simulink model "problem2_4"  (R2020a)
settings: Solver=VariableStepAuto  StartTime=0.0  StopTime=10.0  RelTol=1e-3
settings Model: EnablePacing=on  PacingRate=110  Creator=dinhm  LastModifiedBy=dinhm

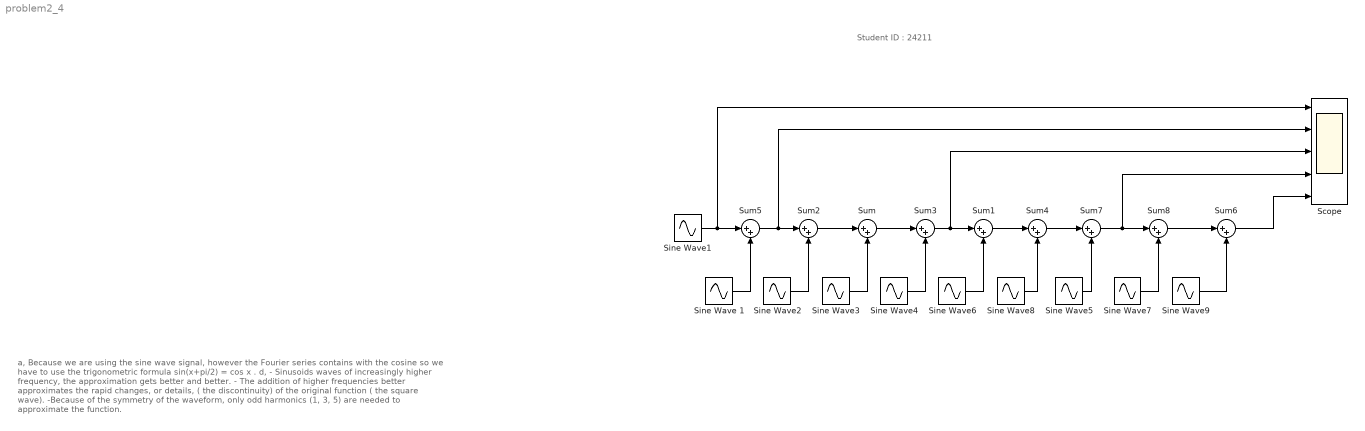
== system problem2_4 ==
  note: a, Because we are using the sine wave signal, however the Fourier series contains with the cosine so we have to use the trigonometric formula sin(x+pi/2) = cos x .
      |
      | d,
      | - Sinusoids waves of increasingly higher frequency, the approximation gets better and better.
      | - The addition of higher frequencies better approximates the rapid changes, or details, ( the discontinuity) of the original function ( the square wave).
      | -Because of the symmetry of the waveform, only odd harmonics (1, 3, 5) are needed to approximate the function.
  note: Student ID : 24211
  Scope : Scope  NumInputPorts=5
  Sine Wave 1 : Sin  Amplitude=4/pi*(-1/3)  Frequency=3*(2*pi/11)  Phase=pi/2  SampleTime=0.1
  Sine Wave1 : Sin  Amplitude=4/pi*1  Frequency=1*(2*pi/11)  Phase=pi/2  SampleTime=0.1
  Sine Wave2 : Sin  Amplitude=4/pi*(1/5)  Frequency=5*(2*pi/11)  Phase=pi/2  SampleTime=0.1
  Sine Wave3 : Sin  Amplitude=4/pi*(-1/7)  Frequency=7*(2*pi/11)  Phase=pi/2  SampleTime=0.1
  Sine Wave4 : Sin  Amplitude=4/pi*(1/9)  Frequency=9*(2*pi/11)  Phase=pi/2  SampleTime=0.1
  Sine Wave5 : Sin  Amplitude=4/pi*(-1/15)  Frequency=15*(2*pi/11)  Phase=pi/2  SampleTime=0.1
  Sine Wave6 : Sin  Amplitude=4/pi*(-1/11)  Frequency=11*(2*pi/11)  Phase=pi/2  SampleTime=0.1
  Sine Wave7 : Sin  Amplitude=4/pi*(1/17)  Frequency=17*(2*pi/11)  Phase=pi/2  SampleTime=0.1
  Sine Wave8 : Sin  Amplitude=4/pi*(1/13)  Frequency=13*(2*pi/11)  Phase=pi/2  SampleTime=0.1
  Sine Wave9 : Sin  Amplitude=4/pi*(-1/19)  Frequency=19*(2*pi/11)  Phase=pi/2  SampleTime=0.1
  Sum{,1..8} (9 alike) : Sum  Inputs=|++
  wires:
  Sine Wave9/1 -> Sum6/2
  Sine Wave7/1 -> Sum8/2
  Sine Wave5/1 -> Sum7/2
  Sine Wave8/1 -> Sum4/2
  Sine Wave6/1 -> Sum1/2
  Sine Wave4/1 -> Sum3/2
  Sine Wave3/1 -> Sum/2
  Sine Wave2/1 -> Sum2/2
  Sum2/1 -> Sum/1
  Sum/1 -> Sum3/1
  Sum1/1 -> Sum4/1
  Sum4/1 -> Sum7/1
  Sum7/1 -> Scope/4, Sum8/1
  Sum8/1 -> Sum6/1
  Sum6/1 -> Scope/5
  Sine Wave1/1 -> Scope/1, Sum5/1
  Sine Wave 1/1 -> Sum5/2
  Sum5/1 -> Scope/2, Sum2/1
  Sum3/1 -> Scope/3, Sum1/1
